simulink model "EcoCAR3_Capstone_P2_LEA_GKN_Enerdel_TheREALone"  (R2014a)
settings: Solver=ode45  StartTime=0.0  StopTime=10.0  RelTol=1e-3
undefined symbols (not defined in the file): chas, DriverControls, EcoCAR3_Lib, eng, eng_plant_init, engine, engine_ratio, env, ENV, fd, gb, gb_ctrl_init, gb_ctrl_trs_init, max_cap, max_cell_curr, motor_ratio, motor_sync_k, motor_sync_Kd, motor_sync_Ki, motor_sync_Kp, num_cell_par, num_cell_series, veh, VEH, veh_plant_init, vpa, vpc, vpc_brake_init, whl, whl_plant_init
libraries: simulink x20
(part 1 of 3)
settings Model: Creator=skumar77  LastModifiedBy=Rashad

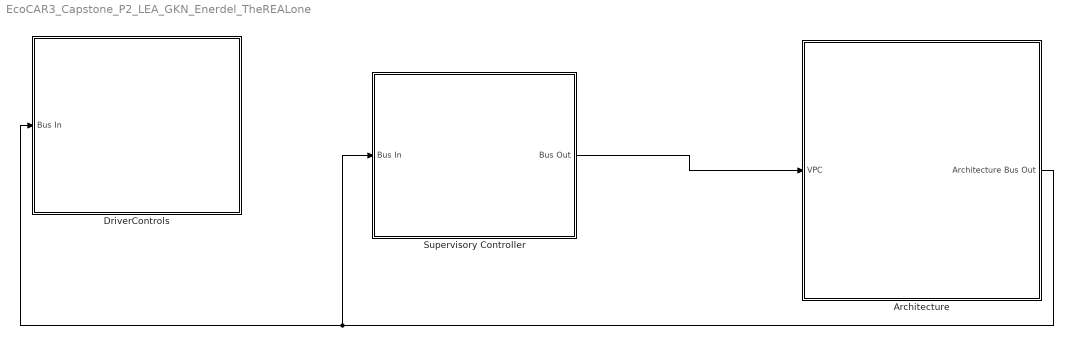
== system EcoCAR3_Capstone_P2_LEA_GKN_Enerdel_TheREALone ==
  Architecture : Subsystem
  DriverControls : Subsystem  AncestorBlock=EcoCAR3_Lib/DriverControls
  Supervisory Controller : Subsystem
  wires:
  Architecture/1(Architecture Bus Out) -> Supervisory Controller/1(Bus In), DriverControls/1(Bus In)
  Supervisory Controller/1(Bus Out) -> Architecture/1(VPC)

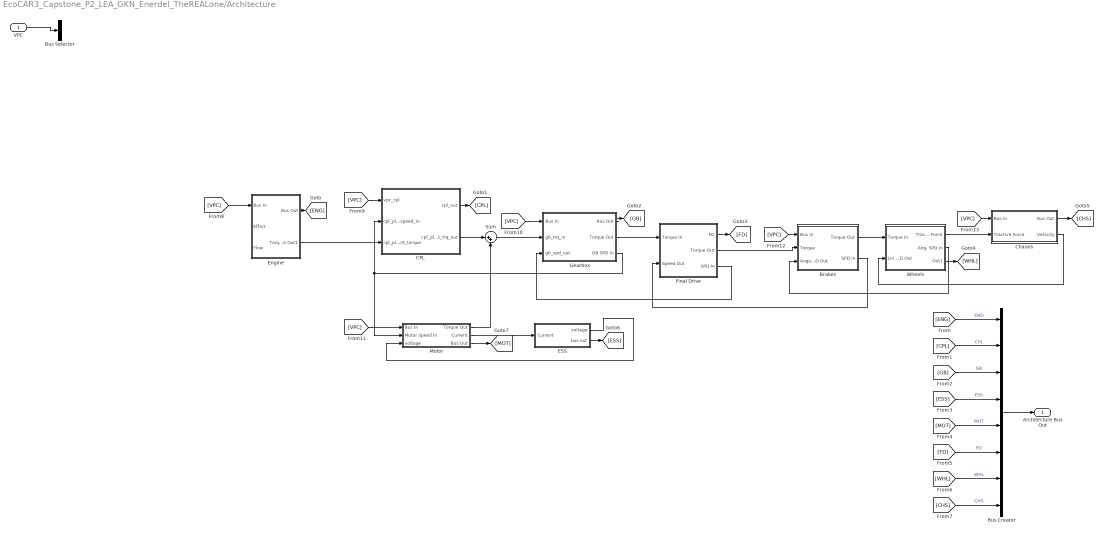
== system EcoCAR3_Capstone_P2_LEA_GKN_Enerdel_TheREALone/Architecture ==
  VPC : Inport
  Brakes : Subsystem
  Bus Creator : BusCreator  Inputs=8
  Bus Selector : BusSelector  OutputSignals=signal1,signal2
  CPL : Subsystem
  Chassis : Subsystem
  ESS : Subsystem
  Engine : Subsystem
  Final Drive : Subsystem
  Gearbox : Subsystem
  Motor : Subsystem
  Sum : Sum  Inputs=|++
  Wheels : Subsystem
  Architecture Bus Out : Outport
  wires:
  Bus Creator/1 -> Architecture Bus Out/1
  [ENG] -> Bus Creator/1  "ENG"
  [CPL] -> Bus Creator/2  "CPL"
  [GB] -> Bus Creator/3  "GB"
  [ESS] -> Bus Creator/4  "ESS"
  [MOT] -> Bus Creator/5  "MOT"
  [FD] -> Bus Creator/6  "FD"
  [WHL] -> Bus Creator/7  "WHL"
  [CHS] -> Bus Creator/8  "CHS"
  Engine/2(Torque Out1) -> CPL/3(cpl_plant_torque)
  Engine/1(Bus Out) -> [ENG]
  Gearbox/3(GB SPD In) -> Motor/2(Motor Speed In), CPL/2(cpl_plant_speed_in)
  Final Drive/3(SPD In) -> Gearbox/3(gb_spd_out)
  Gearbox/2(Torque Out) -> Final Drive/1(Torque In)
  CPL/1(cpl_out) -> [CPL]
  Gearbox/1(Bus Out) -> [GB]
  Final Drive/1(FD) -> [FD]
  CPL/2(cpl_plant_trq_out) -> Sum/1
  Sum/1 -> Gearbox/2(gb_trq_in)
  Motor/1(Torque Out) -> Sum/2
  Final Drive/2(Torque Out) -> Brakes/2(Torque)
  Wheels/2(Ang. SPD In) -> Brakes/3(Angular SPD Out)
  Chassis/2(Velocity) -> Wheels/2(Lin SPD Out)
  Brakes/1(Torque Out) -> Wheels/1(Torque In)
  Brakes/2(SPD In) -> Final Drive/2(Speed Out)
  Wheels/1(Tractive Force) -> Chassis/2(Tractive Force)
  Chassis/1(Bus Out) -> [CHS]
  Motor/2(Current) -> ESS/1(Current)
  ESS/1(voltage) -> Motor/3(voltage)
  Wheels/3(Out1) -> [WHL]
  Motor/3(Bus Out) -> [MOT]
  ESS/2(bus out) -> [ESS]
  [VPC] -> Engine/1(Bus In)
  [VPC] -> CPL/1(vpc_cpl)
  [VPC] -> Gearbox/1(Bus In)
  [VPC] -> Motor/1("Bus In ")
  [VPC] -> Brakes/1(Bus In)
  [VPC] -> Chassis/1(Bus In)
  VPC/1 -> Bus Selector/1

== system EcoCAR3_Capstone_P2_LEA_GKN_Enerdel_TheREALone/DriverControls ==
  Bus In : Inport
  Bus Selector : BusSelector  OutputSignals=CHS
  Driver : Subsystem
  Velocity Profile : Subsystem
  wires:
  Bus Selector/1 -> Driver/2(Measured Velocity)  "<CHS>"
  Velocity Profile/1(Out1) -> Driver/1(Commanded Velocity)
  Bus In/1 -> Bus Selector/1

== system EcoCAR3_Capstone_P2_LEA_GKN_Enerdel_TheREALone/Supervisory Controller ==
  Bus In : Inport
  Brake : Subsystem  Commented=on
  ComponentDiag : Subsystem
  SignalDiag : Subsystem
  Subsystem : Subsystem  Commented=on
  SupervisoryControl : Subsystem
  System Diag : Subsystem
  vpc_prop_par_direct_pwr_1mot_pretx : Subsystem  Commented=on
  Bus Out : Outport
  wires:
  Bus In/1 -> SignalDiag/1(In1)
  SignalDiag/1(Out1) -> ComponentDiag/1(In1)
  ComponentDiag/1(Out1) -> System Diag/1(In1)
  System Diag/1(Out1) -> SupervisoryControl/1(In1)
  SupervisoryControl/1(Out1) -> Bus Out/1

== system EcoCAR3_Capstone_P2_LEA_GKN_Enerdel_TheREALone/Architecture/Brakes ==
  Bus In : Inport
  Torque : Inport  Port=2
  Angular SPD Out : Inport  Port=3
  Plant : Subsystem
  Torque Out : Outport
  SPD In : Outport  Port=2
  wires:
  Torque/1 -> Plant/2(Torque In)
  Angular SPD Out/1 -> Plant/3(Angular Speed Out)
  Plant/2(Angular Speed In) -> SPD In/1
  Plant/1(Torque Out) -> Torque Out/1
  Bus In/1 -> Plant/1(Brake CMD)

== system EcoCAR3_Capstone_P2_LEA_GKN_Enerdel_TheREALone/Architecture/CPL ==
  vpc_cpl : Inport
  cpl_plant_speed_in : Inport  Port=2
  cpl_plant_torque : Inport  Port=3
  Bus Creator : BusCreator  Inputs=2
  Bus Selector : BusSelector  OutputSignals=signal2.cpl_plant_trq_out
  Ctrl : Subsystem
  Plant : Subsystem
  cpl_out : Outport
  cpl_plant_trq_out : Outport  Port=2
  wires:
  Bus Creator/1 -> Bus Selector/1, cpl_out/1
  [PLNT] -> Bus Creator/2
  [CTRL] -> Bus Creator/1
  vpc_cpl/1 -> Ctrl/1(vpc_cpl)
  Ctrl/1(cpl_ctrl_command) -> Plant/1(cpl_command), [CTRL]
  Plant/1(cpl_plant_out) -> [PLNT]
  cpl_plant_torque/1 -> Plant/2(cpl_torque)
  Bus Selector/1 -> cpl_plant_trq_out/1  "<cpl_plant_trq_out>"
  cpl_plant_speed_in/1 -> Plant/3(cpl_speed)

== system EcoCAR3_Capstone_P2_LEA_GKN_Enerdel_TheREALone/Architecture/Chassis ==
  Bus In : Inport
  Tractive Force : Inport  Port=2
  Plant : Subsystem
  Bus Out : Outport
  Velocity : Outport  Port=2
  wires:
  Plant/1(Velocity) -> Velocity/1
  Tractive Force/1 -> Plant/1(Tractive Force)
  Bus In/1 -> Plant/2(Accelerator Position)
  Plant/2(Bus Out) -> Bus Out/1

== system EcoCAR3_Capstone_P2_LEA_GKN_Enerdel_TheREALone/Architecture/ESS ==
  Current : Inport
  Bus Creator : BusCreator  Inputs=3
  Bus Creator1 : BusCreator
  Bus Creator2 : BusCreator  Inputs=2
  Plant : Subsystem
  ess_controller_PI : Subsystem
  voltage : Outport
  bus out : Outport  Port=2
  wires:
  Current/1 -> Bus Creator/1, Plant/1(Current)  "current"
  Plant/2(voltage) -> Bus Creator/2, voltage/1  "voltage"
  Bus Creator/1 -> ess_controller_PI/1(In1)
  ess_controller_PI/4(current_max_reg) -> Bus Creator1/4
  ess_controller_PI/3(power_max_reg) -> Bus Creator1/3
  ess_controller_PI/2(current_max_prop) -> Bus Creator1/2
  ess_controller_PI/1(power_max_prop) -> Bus Creator1/1
  Plant/1("SOC ") -> Bus Creator/3, Bus Creator2/1  "soc"
  Plant/3(bus out) -> Bus Creator2/2
  Bus Creator2/1 -> bus out/1

== system EcoCAR3_Capstone_P2_LEA_GKN_Enerdel_TheREALone/Architecture/Engine ==
  Bus In : Inport
  Effort : Inport  Port=2
  Flow : Inport  Port=3
  Bus Creator : BusCreator  Inputs=2
  Bus Selector : BusSelector  OutputSignals=signal1,signal2
  Controller : Subsystem
  Plant1 : Subsystem
  Bus Out : Outport
  Torque Out1 : Outport  Port=2
  wires:
  Bus Creator/1 -> Bus Out/1
  [CTRL] -> Bus Creator/1  "CTRL"
  [PLNT] -> Bus Creator/2  "PLT"
  Bus In/1 -> Bus Selector/1
  Plant1/1(Bus Out) -> [PLNT]
  Plant1/2(Torque Out) -> Torque Out1/1
  Flow/1 -> Plant1/1(Engine Speed)

== system EcoCAR3_Capstone_P2_LEA_GKN_Enerdel_TheREALone/Architecture/Final Drive ==
  Torque In : Inport
  Speed Out : Inport  Port=2
  Bus Creator : BusCreator  Inputs=1
  Bus Creator1 : BusCreator  Inputs=2
  Plant : Subsystem
  FD : Outport
  Torque Out : Outport  Port=2
  SPD In : Outport  Port=3
  wires:
  Speed Out/1 -> Plant/1(FD SPD Out)
  Torque In/1 -> Plant/2(FD Torque In)
  Plant/1(SPD In) -> Bus Creator1/1, SPD In/1  "gb_plant_spd_in"
  Plant/2(Torque Out) -> Bus Creator1/2, Torque Out/1  "gb_plant_trq_out"
  Bus Creator/1 -> FD/1
  [PLNT] -> Bus Creator/1
  Bus Creator1/1 -> [PLNT]

== system EcoCAR3_Capstone_P2_LEA_GKN_Enerdel_TheREALone/Architecture/Gearbox ==
  Bus In : Inport
  gb_trq_in : Inport  Port=2
  gb_spd_out : Inport  Port=3
  Bus Creator : BusCreator  Inputs=2
  Bus Creator1 : BusCreator  Inputs=2
  Controller : Subsystem
  Plant : Subsystem
  Bus Out : Outport
  Torque Out : Outport  Port=2
  GB SPD In : Outport  Port=3
  wires:
  Controller/1(Out1) -> Plant/3(Gear CMD), [CTRL]
  gb_spd_out/1 -> Plant/1(GB SPD Out)
  gb_trq_in/1 -> Plant/2(GB Torque in)
  Plant/1(GB SPD In) -> Bus Creator1/1, GB SPD In/1  "gb_plant_spd_in"
  Bus Creator/1 -> Bus Out/1
  [CTRL] -> Bus Creator/2
  [PLNT] -> Bus Creator/1
  Plant/2(GB Torque Out) -> Bus Creator1/2, Torque Out/1  "gb_trq_out"
  Bus Creator1/1 -> [PLNT]
  Bus In/1 -> Controller/1(In1)

== system EcoCAR3_Capstone_P2_LEA_GKN_Enerdel_TheREALone/Architecture/Motor ==
  "Bus In " : Inport
  Motor Speed In : Inport  Port=2
  voltage : Inport  Port=3
  Bus Creator : BusCreator  Inputs=2
  Controller : Subsystem
  Plant : Subsystem
  Torque Out : Outport
  Current : Outport  Port=2
  Bus Out : Outport  Port=3
  wires:
  Controller/1(Out1) -> Plant/2(Torque CMD %)
  Motor Speed In/1 -> Plant/1(Motor Speed)
  "Bus In "/1 -> Controller/1(In1)
  Plant/2(Current) -> Current/1
  Plant/1(Torque Out) -> Torque Out/1
  voltage/1 -> Plant/3(voltage)
  [CTRL] -> Bus Creator/2  "CTRL"
  [PLNT] -> Bus Creator/1  "PLNT"
  Bus Creator/1 -> Bus Out/1
  Plant/3(motor_plnt) -> [PLNT]
  Controller/2(bus out) -> [CTRL]

== system EcoCAR3_Capstone_P2_LEA_GKN_Enerdel_TheREALone/Architecture/Wheels ==
  Torque In : Inport
  Lin SPD Out : Inport  Port=2
  Bus Creator : BusCreator  Inputs=2
  Plant : Subsystem
  Tractive Force : Outport
  Ang. SPD In : Outport  Port=2
  Out1 : Outport  Port=3
  wires:
  Torque In/1 -> Plant/1(Wheel Torque)
  Lin SPD Out/1 -> Plant/2(Linear Speed in)
  Plant/1(Tractive Force) -> Bus Creator/1, Tractive Force/1  "whl_plant_tractiveforce"
  Plant/2(Angular Speed) -> Bus Creator/2, Ang. SPD In/1  "whl_plant_speed"
  Bus Creator/1 -> Out1/1

== system EcoCAR3_Capstone_P2_LEA_GKN_Enerdel_TheREALone/DriverControls/Driver ==
  Commanded Velocity : Inport
  Measured Velocity : Inport  Port=2
  BrakeForce : Gain  Gain=5000
  Gain : Gain  Gain=-1
  Memory : Memory
  Memory1 : Memory
  PID Controller : simulink/Continuous/PID Controller  Controller=PI  TimeDomain=Continuous-time  SampleTime=1  IntegratorMethod=Forward Euler  FilterMethod=Forward Euler  Form=Parallel  P=.2  I=.004  D=0  N=100  InitialConditionSource=internal  InitialConditionForIntegrator=0  InitialConditionForFilter=0  ExternalReset=none  LimitOutput=on  UpperSaturationLimit=1  LowerSaturationLimit=-5  LinearizeAsGain=on  AntiWindupMode=clamping  Kb=1  TrackingMode=off  Kt=1  PParamMin=[]  PParamMax=[]  IParamMin=[]  IParamMax=[]  DParamMin=[]  DParamMax=[]  NParamMin=[]  NParamMax=[]  KbParamMin=[]  KbParamMax=[]  KtParamMin=[]  KtParamMax=[]  POutMin=[]  POutMax=[]  IOutMin=[]  IOutMax=[]  DOutMin=[]  DOutMax=[]  NOutMin=[]  NOutMax=[]  KbOutMin=[]  KbOutMax=[]  KtOutMin=[]  KtOutMax=[]  IntegratorOutMin=[]  IntegratorOutMax=[]  FilterOutMin=[]  FilterOutMax=[]  SumOutMin=[]  SumOutMax=[]  SumI1OutMin=[]  SumI1OutMax=[]  SumI2OutMin=[]  SumI2OutMax=[]  SumI3OutMin=[]  SumI3OutMax=[]  SumDOutMin=[]  SumDOutMax=[]  SaturationOutMin=[]  SaturationOutMax=[]  IntegratorContinuousStateAttributes=''  IntegratorStateMustResolveToSignalObject=off  IntegratorRTWStateStorageClass=Auto  FilterContinuousStateAttributes=''  FilterStateMustResolveToSignalObject=off  FilterRTWStateStorageClass=Auto
  Pct : Gain  Gain=100
  Saturation : Saturate  UpperLimit=1  LowerLimit=0
  Saturation1 : Saturate  UpperLimit=0  LowerLimit=-1
  Sum1 : Sum  Inputs=+-|
  Brake : Outport
  Accelerator Position : Outport  Port=2
  wires:
  Commanded Velocity/1 -> Sum1/2
  Sum1/1 -> PID Controller/1
  Measured Velocity/1 -> Sum1/1
  Pct/1 -> Memory1/1
  Memory/1 -> Brake/1
  Memory1/1 -> Accelerator Position/1
  BrakeForce/1 -> Memory/1
  Saturation/1 -> BrakeForce/1
  PID Controller/1 -> Saturation/1, Saturation1/1
  Saturation1/1 -> Gain/1
  Gain/1 -> Pct/1

== system EcoCAR3_Capstone_P2_LEA_GKN_Enerdel_TheREALone/DriverControls/Velocity Profile ==
  DriveCycle Select : Subsystem  AncestorBlock=EcoCAR3_Lib/DriveCycle Select  mask(Drive Cycle){Drive_Cycle_Num=EcoCAR city 1}
      mask prompts: Drive_Cycle_Num "Select the desired drive cycle"
      mask help:
      | Select the drive cycle you wish to input to the vehicle model.
      | The simulation run time and assertions will be updated accordingly.
      settings: AttributesFormatString=%<Drive_Cycle_Num> (kph)
      mask TypeOptions Drive_Cycle_Num: EcoCAR city 1 | EcoCAR city 2 | EcoCAR hwy | FTP75 | Cruise Mode | US06
      mask Callback Drive_Cycle_Num:
      | maskStr = get_param(gcb,'MaskValues');
      | maskStr = maskStr{1};
      | mdnm = get_param(gcs,'Name');
      | % Urban 1
      | % Urban 2
      | % Urban 3
      | % Urban 4
      | % FTP75
      | % US06
      | % Combined 0-60, FTP75
      | % Combined 0-60, US06
      | switch maskStr
      |     case 'Urban 1'
      |         setsim(1,200,mdnm);
      |         zero2sixty_cuttoff_time = inf;
      |     case 'Urban 2'
      |         setsim(2,200,mdnm);
      |         zero2sixty_cuttoff_time = inf;
      |     case 'Urban 3'
      |         setsim(3,200,mdnm);
      |         zero2sixty_cuttoff_time = inf;
      |     case 'FTP75'
      |         setsim(4,490,mdnm);
      |         zero2sixty_cuttoff_time = inf;
      |     case 'Cruise Mode'
      |         setsim(5,129,mdnm);
      |         zero2sixty_cuttoff_time = inf;
      |     case 'US06'
      |         setsim(6,600,mdnm);
      |         zero2sixty_cuttoff_time = inf;
      |     case 'Combined 0-60, FTP75'
      |         setsim(7,650,mdnm);
      |         zero2sixty_cuttoff_time = 15;
      |     case 'Combined 0-60, US06'
      |         setsim(8,650,mdnm);
      |         zero2sixty_cuttoff_time = 15;
      |     otherwise
      |         setsim(8,650,mdnm);
      |         zero2sixty_cuttoff_time = 15;
      | end
      | 
      | % function setsim(caseno,simtime,modelname)
      | %      assignin('base','Drive_Cycle_Num',caseno);
      | %      evalin('base',['set_param(''' modelname ''',''StartTime'',''0'',''StopTime'',''' num2str(simtime) ''') ';'']);
      | %      %eval(['set_param(''' modelname ''',''StartTime'',''0'',''StopTime'',''' num2str(simtime) ''') ';'']);
      | % end
  Subsystem : Subsystem  mask(Select Mode){Choice=DriveCycle Select}
      mask prompts: Choice "Select mode"
      mask help: Select acceleration, braking or drive cycle execution mode
      mask TypeOptions Choice: acceleration test | brake test | DriveCycle Select
  acceleration test : FromWorkspace  VariableName=[acc.time acc.SpdKph]  SampleTime=0
  brake test : FromWorkspace  VariableName=[brake.time brake.SpdKph]  SampleTime=0
  Out1 : Outport
  wires:
  DriveCycle Select/1(kph) -> Subsystem/3(In3)
  brake test/1 -> Subsystem/2(In2)
  acceleration test/1 -> Subsystem/1(In1)
  Subsystem/1(Out1) -> Out1/1  "Velocity Profile"

== system EcoCAR3_Capstone_P2_LEA_GKN_Enerdel_TheREALone/Supervisory Controller/Brake ==
  drv_brk_cmd : Inport
  chas_spd : Inport  Port=2
  ess_soc : Inport  Port=3
  gb_gear_ratio : Inport  Port=4
  gb_gear_sft_in_progress : Inport  Port=5
  cpl_cmd : Inport  Port=6
  mot_main_spd : Inport  Port=7
  ess_pwr_max_neg : Inport  Port=8
  mot_main_trq_max : Inport  Port=9
  Brake ECU Torque : Subsystem
  Chassis speed ESS SOC limits : Subsystem
  Electric power available : Subsystem
  Gear shifting : Subsystem
  Main motor brake torque demand : Subsystem
  Motor main torque max : Subsystem
  Saturation : Saturate  UpperLimit=0  LowerLimit=-inf
  Sum : Sum  Inputs=+-
  Terminator : Terminator
  Terminator1 : Terminator
  "Torque demand at wheels " : Subsystem
  whl_brk_trq_ECU_dmd : Outport
  mot_main_trq_dmd : Outport  Port=2
  wires:
  drv_brk_cmd/1 -> "Torque demand at wheels "/1(brake_signal_dmd)
  "Torque demand at wheels "/1(whl_trq_dmd) -> Brake ECU Torque/1(whl_trq_dmd)
  Brake ECU Torque/2(whl_twr_brk_ECU) -> Chassis speed ESS SOC limits/1(whl_trq_brake_ECU), Sum/1
  Brake ECU Torque/1(whl_twr_brk_emergency) -> Terminator/1
  Sum/1 -> Saturation/1
  Saturation/1 -> whl_brk_trq_ECU_dmd/1
  ess_soc/1 -> Chassis speed ESS SOC limits/3(ess_soc)
  Chassis speed ESS SOC limits/1(whl_trq_regen_available) -> Main motor brake torque demand/1(whl_trq_regen_max)
  Main motor brake torque demand/1(mot_trq_dmd) -> mot_main_trq_dmd/1
  Main motor brake torque demand/3(mot_pwr_elec_estimated) -> Terminator1/1
  Main motor brake torque demand/2(mot_trq_dmd_at_wheels) -> Sum/2
  gb_gear_ratio/1 -> Gear shifting/1(gb_gear_ratio)
  gb_gear_sft_in_progress/1 -> Gear shifting/2(gb_sft_in_progress)
  cpl_cmd/1 -> Gear shifting/3(cpl_cmd)
  Gear shifting/1(gear_ratio) -> Main motor brake torque demand/2(ratio_gear)
  Gear shifting/2(coeff_mult_gear) -> Main motor brake torque demand/3(coef_mult_sft)
  ess_pwr_max_neg/1 -> Electric power available/1(ess_pwr_max_neg)
  Electric power available/1(pwr_elec_available_regen) -> Motor main torque max/2(pwr_elec_max)
  mot_main_spd/1 -> Motor main torque max/1(mot_spd), Main motor brake torque demand/4(mot_spd)
  mot_main_trq_max/1 -> Motor main torque max/3(mot_trq_max)
  Motor main torque max/1(mot_trq_maximum) -> Main motor brake torque demand/5(mot_trq_max_regen)
  chas_spd/1 -> Chassis speed ESS SOC limits/2(chas_spd)

== system EcoCAR3_Capstone_P2_LEA_GKN_Enerdel_TheREALone/Supervisory Controller/ComponentDiag ==
  In1 : Inport
  Bus Creator{,1..5} (6 alike) : BusCreator  Inputs=2
  Bus Selector{,1..5} (6 alike) : BusSelector  OutputSignals=signal1,signal2
  Out1 : Outport
  wires:
  In1/1 -> Bus Selector5/1, Bus Selector4/1, Bus Selector3/1, Bus Selector2/1, Bus Selector1/1, Bus Selector/1

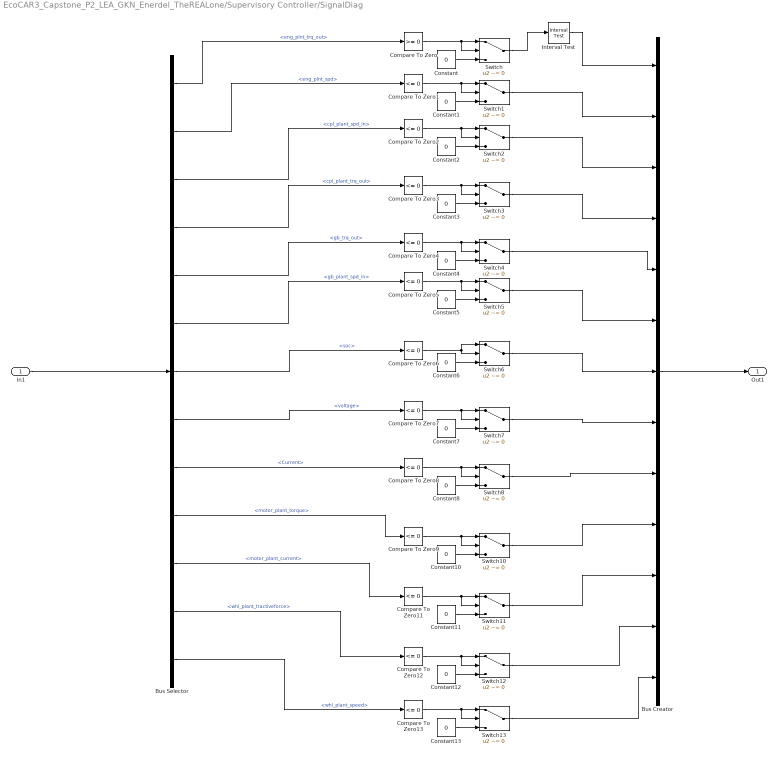
== system EcoCAR3_Capstone_P2_LEA_GKN_Enerdel_TheREALone/Supervisory Controller/SignalDiag ==
  In1 : Inport
  Bus Creator : BusCreator  Inputs=13
  Bus Selector : BusSelector  OutputSignals=ENG.PLT.eng_plnt_trq_out,ENG.PLT.eng_plnt_spd,CPL.signal2.cpl_plant_spd_in,CPL.signal2.cpl_plant_trq_out,GB.signal1.gb_trq_out,GB.signal1.gb_plant_spd_in,ESS.soc,ESS.signal2.voltage,ESS.signal2.Current,MOT.PLNT.motor_plant_torque,MOT.PLNT.motor_plant_current,WHL.whl_plant_tractiveforce,WHL.whl_plant_speed
  Compare To Zero : simulink/Logic and Bit Operations/Compare To Zero  relop=>=  OutDataTypeStr=boolean
  Compare To Zero{1..9,11..13} (12 alike) : simulink/Logic and Bit Operations/Compare To Zero  relop=<=  OutDataTypeStr=boolean
  Constant{,1..8,10..13} (13 alike) : Constant  Value=0
  Interval Test : simulink/Logic and Bit Operations/Interval Test  IntervalClosedRight=on  uplimit=0.5  IntervalClosedLeft=on  lowlimit=-0.5  OutDataTypeStr=boolean
  Switch{,1..8,10..13} (13 alike) : Switch  Criteria=u2 ~= 0
  Out1 : Outport
  wires:
  In1/1 -> Bus Selector/1
  Bus Creator/1 -> Out1/1
  Compare To Zero/1 -> Switch/2, Switch/1
  Constant/1 -> Switch/3
  Compare To Zero1/1 -> Switch1/1, Switch1/2
  Constant1/1 -> Switch1/3
  Compare To Zero2/1 -> Switch2/2, Switch2/1
  Constant2/1 -> Switch2/3
  Compare To Zero3/1 -> Switch3/1, Switch3/2
  Constant3/1 -> Switch3/3
  Compare To Zero4/1 -> Switch4/2, Switch4/1
  Constant4/1 -> Switch4/3
  Compare To Zero5/1 -> Switch5/1, Switch5/2
  Constant5/1 -> Switch5/3
  Compare To Zero6/1 -> Switch6/1, Switch6/2
  Constant6/1 -> Switch6/3
  Compare To Zero7/1 -> Switch7/1, Switch7/2
  Constant7/1 -> Switch7/3
  Compare To Zero8/1 -> Switch8/2, Switch8/1
  Constant8/1 -> Switch8/3
  Compare To Zero9/1 -> Switch10/2, Switch10/1
  Constant10/1 -> Switch10/3
  Compare To Zero11/1 -> Switch11/1, Switch11/2
  Constant11/1 -> Switch11/3
  Compare To Zero12/1 -> Switch12/2, Switch12/1
  Constant12/1 -> Switch12/3
  Compare To Zero13/1 -> Switch13/1, Switch13/2
  Constant13/1 -> Switch13/3
  Bus Selector/13 -> Compare To Zero13/1  "<whl_plant_speed>"
  Bus Selector/12 -> Compare To Zero12/1  "<whl_plant_tractiveforce>"
  Bus Selector/11 -> Compare To Zero11/1  "<motor_plant_current>"
  Bus Selector/10 -> Compare To Zero9/1  "<motor_plant_torque>"
  Bus Selector/9 -> Compare To Zero8/1  "<Current>"
  Bus Selector/8 -> Compare To Zero7/1  "<voltage>"
  Bus Selector/7 -> Compare To Zero6/1  "<soc>"
  Bus Selector/6 -> Compare To Zero5/1  "<gb_plant_spd_in>"
  Bus Selector/5 -> Compare To Zero4/1  "<gb_trq_out>"
  Bus Selector/4 -> Compare To Zero3/1  "<cpl_plant_trq_out>"
  Bus Selector/3 -> Compare To Zero2/1  "<cpl_plant_spd_in>"
  Bus Selector/2 -> Compare To Zero1/1  "<eng_plnt_spd>"
  Bus Selector/1 -> Compare To Zero/1  "<eng_plnt_trq_out>"
  Switch8/1 -> Bus Creator/9
  Switch7/1 -> Bus Creator/8
  Switch6/1 -> Bus Creator/7
  Switch5/1 -> Bus Creator/6
  Switch4/1 -> Bus Creator/5
  Switch3/1 -> Bus Creator/4
  Switch2/1 -> Bus Creator/3
  Switch1/1 -> Bus Creator/2
  Switch/1 -> Interval Test/1
  Switch10/1 -> Bus Creator/10
  Switch11/1 -> Bus Creator/11
  Switch12/1 -> Bus Creator/12
  Switch13/1 -> Bus Creator/13
  Interval Test/1 -> Bus Creator/1

== system EcoCAR3_Capstone_P2_LEA_GKN_Enerdel_TheREALone/Supervisory Controller/Subsystem ==
  Eng : Inport
  ESS : Inport  Port=2
  CPL : Inport  Port=3
  Motor : Inport  Port=4
  GB : Inport  Port=5
  FD : Inport  Port=6
  WHL : Inport  Port=7
  CHS : Inport  Port=8
  Key pos : Inport  Port=9
  Constant : Constant  Value=0
  Rate Limiter2 : RateLimiter  RisingSlewLimit=250  FallingSlewLimit=-250  SampleTimeMode=inherited
  SupervisoryLogicChart : Stateflow chart  TreatAsAtomicUnit=on
  VPC Eng : Outport
  "VPC CPL " : Outport  Port=2
  VPC motor : Outport  Port=3
  VPC GB : Outport  Port=4
  VPC Brakes : Outport  Port=5
  VPC CHS : Outport  Port=6
  wires:
  ? -> SupervisoryLogicChart/1(eSystemStatus)  "<eSystemStatus>"
  ? -> SupervisoryLogicChart/3(APP_percent)  "<APP [%]>"
  ? -> SupervisoryLogicChart/4(BPP_percent)  "<BPP [%]>"
  ? -> SupervisoryLogicChart/5(keyPos)  "< keyPos [0_3]>"
  SupervisoryLogicChart/1(motTrqReq_percent) -> Rate Limiter2/1
  SupervisoryLogicChart/7(ChartMode) -> ?
  ? -> SupervisoryLogicChart/6(vehVel_mph)  "<vehVel [mph]>"
  SupervisoryLogicChart/3(hydBrkReq_percent) -> ?
  ? -> SupervisoryLogicChart/7(regenFactor)  "<regenFactor>"
  ? -> ?  "<PRNDL>"
  SupervisoryLogicChart/2(engTrqReq_percent) -> ?
  SupervisoryLogicChart/4(powerMode) -> ?
  SupervisoryLogicChart/5(closeContactorsReq) -> ?
  SupervisoryLogicChart/6(engOnReq) -> ?
  ? -> SupervisoryLogicChart/2(iceSystemStatus)  "<iceSystemStatus>"
  Rate Limiter2/1 -> ?  "motTrqReq_percent"
  Constant/1 -> SupervisoryLogicChart/9(motDrag_percent)
  ? -> SupervisoryLogicChart/8(essSOC_0_1)  "<essSOC_0_1>"

== system EcoCAR3_Capstone_P2_LEA_GKN_Enerdel_TheREALone/Supervisory Controller/SupervisoryControl ==
  In1 : Inport
  Bus Creator : BusCreator  Inputs=2
  Bus Selector : BusSelector  OutputSignals=signal1,signal2
  SupervisorLogic : Stateflow chart  TreatAsAtomicUnit=on
  Out1 : Outport
  wires:
  In1/1 -> Bus Selector/1
  Bus Creator/1 -> Out1/1

== system EcoCAR3_Capstone_P2_LEA_GKN_Enerdel_TheREALone/Supervisory Controller/System Diag ==
  In1 : Inport
  Bus Creator{,1..3} (4 alike) : BusCreator  Inputs=2
  Bus Selector{,1..3} (4 alike) : BusSelector  OutputSignals=signal1,signal2
  Out1 : Outport

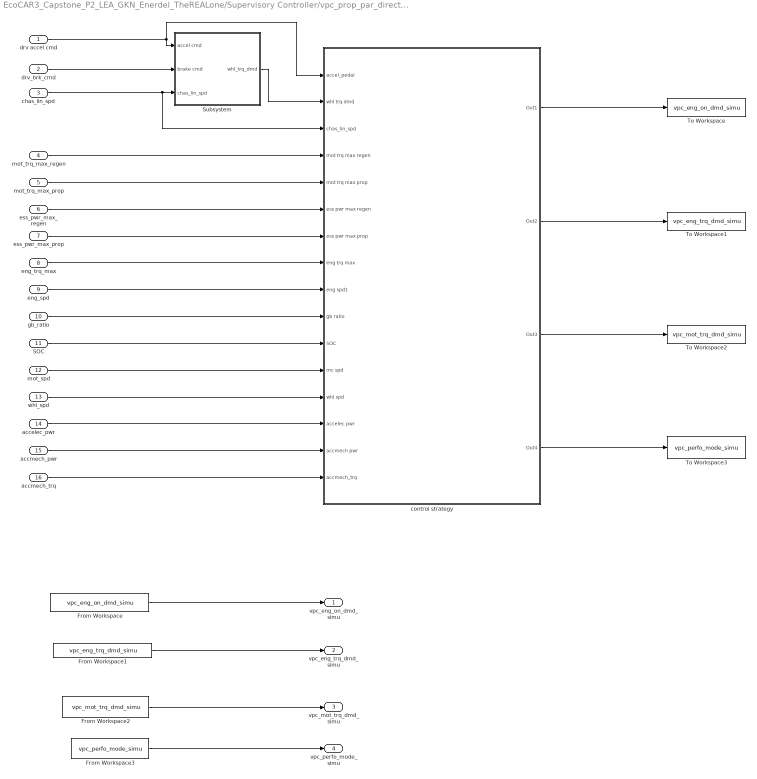
== system EcoCAR3_Capstone_P2_LEA_GKN_Enerdel_TheREALone/Supervisory Controller/vpc_prop_par_direct_pwr_1mot_pretx ==
  drv accel cmd : Inport
  drv_brk_cmd : Inport  Port=2
  chas_lin_spd : Inport  Port=3
  mot_trq_max_regen : Inport  Port=4
  mot_trq_max_prop : Inport  Port=5
  ess_pwr_max_regen : Inport  Port=6
  ess_pwr_max_prop : Inport  Port=7
  eng_trq_max : Inport  Port=8
  eng_spd : Inport  Port=9
  gb_ratio : Inport  Port=10
  SOC : Inport  Port=11
  mot_spd : Inport  Port=12
  whl_spd : Inport  Port=13
  accelec_pwr : Inport  Port=14
  accmech_pwr : Inport  Port=15
  accmech_trq : Inport  Port=16
  From Workspace : FromWorkspace  VariableName=vpc_eng_on_dmd_simu  SampleTime=0
  From Workspace1 : FromWorkspace  VariableName=vpc_eng_trq_dmd_simu  SampleTime=0
  From Workspace2 : FromWorkspace  VariableName=vpc_mot_trq_dmd_simu  SampleTime=0
  From Workspace3 : FromWorkspace  VariableName=vpc_perfo_mode_simu  SampleTime=0
  Subsystem : Subsystem
  To Workspace : ToWorkspace  VariableName=vpc_eng_on_dmd_simu  SaveFormat=Timeseries  SampleTime=-1
  To Workspace1 : ToWorkspace  VariableName=vpc_eng_trq_dmd_simu  SaveFormat=Timeseries  SampleTime=-1
  To Workspace2 : ToWorkspace  VariableName=vpc_mot_trq_dmd_simu  SaveFormat=Timeseries  SampleTime=-1
  To Workspace3 : ToWorkspace  VariableName=vpc_perfo_mode_simu  SaveFormat=Timeseries  SampleTime=-1
  control strategy : Subsystem
  vpc_eng_on_dmd_simu : Outport
  vpc_eng_trq_dmd_simu : Outport  Port=2
  vpc_mot_trq_dmd_simu : Outport  Port=3
  vpc_perfo_mode_simu : Outport  Port=4
  wires:
  From Workspace2/1 -> vpc_mot_trq_dmd_simu/1
  From Workspace1/1 -> vpc_eng_trq_dmd_simu/1
  From Workspace/1 -> vpc_eng_on_dmd_simu/1
  From Workspace3/1 -> vpc_perfo_mode_simu/1
  drv_brk_cmd/1 -> Subsystem/2(brake cmd)
  chas_lin_spd/1 -> control strategy/3(chas_lin_spd), Subsystem/3(chas_lin_spd)
  drv accel cmd/1 -> Subsystem/1(accel cmd), control strategy/1(accel_pedal)
  Subsystem/1(whl_trq_dmd) -> control strategy/2(whl trq dmd)
  mot_trq_max_regen/1 -> control strategy/4(mot trq max regen)
  mot_trq_max_prop/1 -> control strategy/5(mot trq max prop)
  accmech_trq/1 -> control strategy/16(accmech_trq)
  accmech_pwr/1 -> control strategy/15(accmech pwr)
  accelec_pwr/1 -> control strategy/14(accelec pwr)
  whl_spd/1 -> control strategy/13(whl spd)
  ess_pwr_max_regen/1 -> control strategy/6(ess pwr max regen)
  ess_pwr_max_prop/1 -> control strategy/7(ess pwr max prop)
  eng_trq_max/1 -> control strategy/8(eng trq max)
  eng_spd/1 -> control strategy/9(eng spd1)
  gb_ratio/1 -> control strategy/10(gb ratio)
  SOC/1 -> control strategy/11(SOC)
  mot_spd/1 -> control strategy/12(mc spd)
  control strategy/4(Out4) -> To Workspace3/1
  control strategy/3(Out3) -> To Workspace2/1
  control strategy/2(Out2) -> To Workspace1/1
  control strategy/1(Out1) -> To Workspace/1

== system EcoCAR3_Capstone_P2_LEA_GKN_Enerdel_TheREALone/Architecture/Brakes/Plant ==
  Brake CMD : Inport
  Torque In : Inport  Port=2
  Angular Speed Out : Inport  Port=3
  Max Brake Force : Constant  Value=whl.brake.max_force
  Product : Product
  Subtract : Sum  Inputs=-+
  Torque Out : Outport
  Angular Speed In : Outport  Port=2
  wires:
  Angular Speed Out/1 -> Angular Speed In/1
  Max Brake Force/1 -> Product/2
  Product/1 -> Subtract/1
  Subtract/1 -> Torque Out/1
  Brake CMD/1 -> Product/1
  Torque In/1 -> Subtract/2

== system EcoCAR3_Capstone_P2_LEA_GKN_Enerdel_TheREALone/Architecture/CPL/Ctrl ==
  vpc_cpl : Inport
  Constant1 : Constant
  Constant2 : Constant  Value=0
  Index Vector : MultiPortSwitch  DataPortOrder=Zero-based contiguous  zeroidx=on
  Rate Limiter : RateLimiter  RisingSlewLimit=2.5  SampleTimeMode=inherited
  Saturation : Saturate  UpperLimit=1  LowerLimit=0
  cpl_ctrl_command : Outport
  wires:
  Index Vector/1 -> cpl_ctrl_command/1
  vpc_cpl/1 -> Index Vector/1, Rate Limiter/1
  Saturation/1 -> Index Vector/4
  Constant2/1 -> Index Vector/2
  Constant1/1 -> Index Vector/3
  Rate Limiter/1 -> Saturation/1

== system EcoCAR3_Capstone_P2_LEA_GKN_Enerdel_TheREALone/Architecture/CPL/Plant ==
  cpl_command : Inport
  cpl_torque : Inport  Port=2
  cpl_speed : Inport  Port=3
  Bus Creator : BusCreator  Inputs=2
  Product : Product
  Product1 : Product
  cpl_plant_out : Outport
  wires:
  cpl_torque/1 -> Product1/2
  cpl_command/1 -> Product1/1, Product/2
  Product1/1 -> Bus Creator/2  "cpl_plant_trq_out"
  Product/1 -> Bus Creator/1  "cpl_plant_spd_in"
  Bus Creator/1 -> cpl_plant_out/1
  cpl_speed/1 -> Product/1

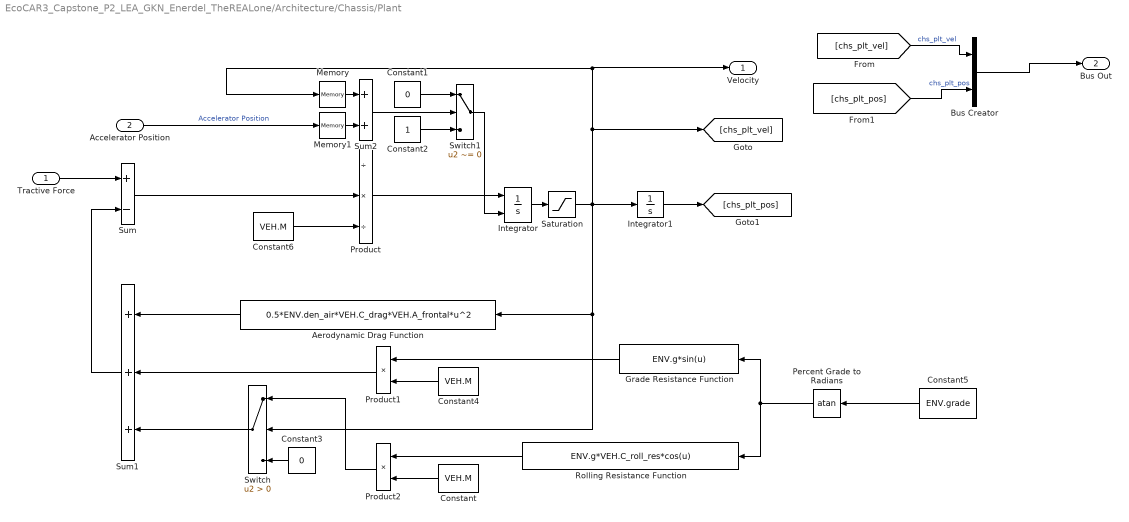
== system EcoCAR3_Capstone_P2_LEA_GKN_Enerdel_TheREALone/Architecture/Chassis/Plant ==
  Tractive Force : Inport
  Accelerator Position : Inport  Port=2
  Aerodynamic Drag Function : Fcn  Expr=0.5*ENV.den_air*VEH.C_drag*VEH.A_frontal*u^2
  Bus Creator : BusCreator  Inputs=2
  Constant : Constant  Value=VEH.M
  Constant1 : Constant  Value=0
  Constant2 : Constant
  Constant3 : Constant  Value=0
  Constant4 : Constant  Value=VEH.M
  Constant5 : Constant  Value=ENV.grade
  Constant6 : Constant  Value=VEH.M
  Grade Resistance Function : Fcn  Expr=ENV.g*sin(u)
  Integrator : Integrator  ExternalReset=level  LowerSaturationLimit=0
  Integrator1 : Integrator
  Memory : Memory
  Memory1 : Memory
  Percent Grade to Radians : Trigonometry  Operator=atan
  Product : Product  Inputs=/*/  RndMeth=Zero
  Product1 : Product  Inputs=**  RndMeth=Zero
  Product2 : Product  Inputs=**  RndMeth=Zero
  Rolling Resistance Function : Fcn  Expr=ENV.g*VEH.C_roll_res*cos(u)
  Saturation : Saturate  UpperLimit=inf  LowerLimit=0
  Sum : Sum  Inputs=+-  SaturateOnIntegerOverflow=on  InputSameDT=on  OutDataTypeStr=Inherit: Same as first input
  Sum1 : Sum  Inputs=+++  SaturateOnIntegerOverflow=on  InputSameDT=on  OutDataTypeStr=Inherit: Same as first input
  Sum2 : Sum  SaturateOnIntegerOverflow=on  InputSameDT=on  OutDataTypeStr=Inherit: Same as first input
  Switch : Switch  Criteria=u2 > Threshold  SaturateOnIntegerOverflow=on  InputSameDT=on
  Switch1 : Switch  Criteria=u2 ~= 0  SaturateOnIntegerOverflow=on  InputSameDT=on
  Velocity : Outport
  Bus Out : Outport  Port=2
  wires:
  Sum1/1 -> Sum/2
  Tractive Force/1 -> Sum/1
  Aerodynamic Drag Function/1 -> Sum1/1
  Integrator1/1 -> [chs_plt_pos]
  Constant3/1 -> Switch/3
  Sum/1 -> Product/2
  Integrator/1 -> Saturation/1
  Switch/1 -> Sum1/3
  Constant5/1 -> Percent Grade to Radians/1
  Percent Grade to Radians/1 -> Rolling Resistance Function/1, Grade Resistance Function/1
  Product/1 -> Integrator/1
  Saturation/1 -> Memory/1, Velocity/1, [chs_plt_vel], Integrator1/1, Switch/2, Aerodynamic Drag Function/1
  Accelerator Position/1 -> Memory1/1  "Accelerator Position"
  Sum2/1 -> Switch1/2
  Switch1/1 -> Integrator/2
  Constant1/1 -> Switch1/1
  Constant2/1 -> Switch1/3
  Memory1/1 -> Sum2/2
  Memory/1 -> Sum2/1
  Constant6/1 -> Product/3
  Grade Resistance Function/1 -> Product1/1
  Product1/1 -> Sum1/2
  Constant4/1 -> Product1/2
  Constant/1 -> Product2/2
  Rolling Resistance Function/1 -> Product2/1
  Product2/1 -> Switch/1
  [chs_plt_vel] -> Bus Creator/1  "chs_plt_vel"
  [chs_plt_pos] -> Bus Creator/2  "chs_plt_pos"
  Bus Creator/1 -> Bus Out/1

== system EcoCAR3_Capstone_P2_LEA_GKN_Enerdel_TheREALone/Architecture/ESS/Plant ==
  Current : Inport
  1/num_cell_par : Gain  Gain=1/num_cell_par
  1/num_cell_par1 : Gain  Gain=1/num_cell_par
  Bus Creator : BusCreator
  SOC Calculation : Subsystem
  Voltage Calculation : Subsystem
  num_cell_series : Gain  Gain=num_cell_series
  num_cell_series1 : Gain  Gain=num_cell_series
  num_cell_series2 : Gain  Gain=num_cell_series
  "SOC " : Outport
  voltage : Outport  Port=2
  bus out : Outport  Port=3
  wires:
  Current/1 -> 1/num_cell_par/1
  SOC Calculation/1(SOC) -> Voltage Calculation/1(SOC), "SOC "/1
  1/num_cell_par/1 -> Voltage Calculation/2(Current), Bus Creator/4, SOC Calculation/1(Current)  "Current"
  Voltage Calculation/1(Open Circuit Voltage) -> num_cell_series/1
  Voltage Calculation/2(Voltage) -> num_cell_series1/1
  num_cell_series1/1 -> Bus Creator/2, voltage/1  "voltage"
  num_cell_series/1 -> Bus Creator/1  "voc"
  Voltage Calculation/3(Internal Resistance) -> num_cell_series2/1
  num_cell_series2/1 -> 1/num_cell_par1/1
  1/num_cell_par1/1 -> Bus Creator/3  "rint"
  Bus Creator/1 -> bus out/1

== system EcoCAR3_Capstone_P2_LEA_GKN_Enerdel_TheREALone/Architecture/ESS/ess_controller_PI ==
  In1 : Inport
  Bus Selector : BusSelector  OutputSignals=current,voltage,soc
  Controller : Subsystem
  Controller1 : Subsystem
  power_max_prop : Outport
  current_max_prop : Outport  Port=2
  power_max_reg : Outport  Port=3
  current_max_reg : Outport  Port=4
  wires:
  Bus Selector/3 -> Controller/3(SOC), Controller1/3(SOC)  "<soc>"
  Bus Selector/2 -> Controller/2(Voltage), Controller1/2(Voltage)  "<voltage>"
  Bus Selector/1 -> Controller1/1(Current), Controller1/4(Current1), Controller/4(Current1), Controller/1(Current)  "<current>"
  In1/1 -> Bus Selector/1
  Controller1/1(power_max_reg) -> power_max_reg/1  "power_max_reg"
  Controller/2(current_max_prop) -> current_max_prop/1  "current_max_prop"
  Controller1/2(current_max_reg) -> current_max_reg/1  "current_max_reg"
  Controller/1(power_max_prop) -> power_max_prop/1  "power_max_prop"

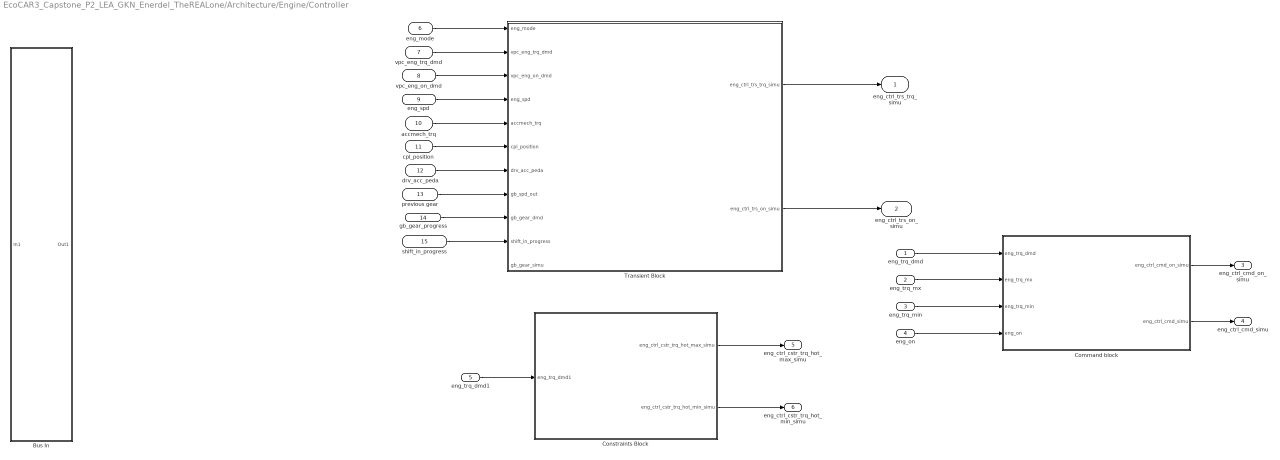
== system EcoCAR3_Capstone_P2_LEA_GKN_Enerdel_TheREALone/Architecture/Engine/Controller ==
  eng_trq_dmd : Inport
  eng_trq_mx : Inport  Port=2
  eng_trq_min : Inport  Port=3
  eng_on : Inport  Port=4
  eng_trq_dmd1 : Inport  Port=5
  eng_mode : Inport  Port=6
  vpc_eng_trq_dmd : Inport  Port=7
  vpc_eng_on_dmd : Inport  Port=8
  eng_spd : Inport  Port=9
  accmech_trq : Inport  Port=10
  cpl_position : Inport  Port=11
  drv_acc_peda : Inport  Port=12
  previous gear : Inport  Port=13
  gb_gear_progress : Inport  Port=14
  shift_in_progress : Inport  Port=15
  Bus In : Subsystem
  "Command block " : Subsystem
  Constraints Block : Subsystem
  Transient Block : Subsystem
  eng_ctrl_trs_trq_simu : Outport
  eng_ctrl_trs_on_simu : Outport  Port=2
  eng_ctrl_cmd_on_simu : Outport  Port=3
  eng_ctrl_cmd_simu : Outport  Port=4
  eng_ctrl_cstr_trq_hot_max_simu : Outport  Port=5
  eng_ctrl_cstr_trq_hot_min_simu : Outport  Port=6
  wires:
  eng_trq_dmd1/1 -> Constraints Block/1(eng_trq_dmd1)
  Constraints Block/1(eng_ctrl_cstr_trq_hot_max_simu) -> eng_ctrl_cstr_trq_hot_max_simu/1
  Constraints Block/2(eng_ctrl_cstr_trq_hot_min_simu) -> eng_ctrl_cstr_trq_hot_min_simu/1
  eng_trq_dmd/1 -> "Command block "/1(eng_trq_dmd)
  eng_trq_mx/1 -> "Command block "/2(eng_trq_mx)
  eng_trq_min/1 -> "Command block "/3(eng_trq_min)
  eng_on/1 -> "Command block "/4(eng_on)
  "Command block "/1(eng_ctrl_cmd_on_simu) -> eng_ctrl_cmd_on_simu/1
  "Command block "/2(eng_ctrl_cmd_simu) -> eng_ctrl_cmd_simu/1
  eng_mode/1 -> Transient Block/1(eng_mode)
  vpc_eng_trq_dmd/1 -> Transient Block/2(vpc_eng_trq_dmd)
  vpc_eng_on_dmd/1 -> Transient Block/3(vpc_eng_on_dmd)
  eng_spd/1 -> Transient Block/4(eng_spd)
  accmech_trq/1 -> Transient Block/5(accmech_trq)
  cpl_position/1 -> Transient Block/6(cpl_position)
  drv_acc_peda/1 -> Transient Block/7(drv_acc_peda)
  previous gear/1 -> Transient Block/8(gb_spd_out)
  shift_in_progress/1 -> Transient Block/10(shift_in_progress)
  Transient Block/1(eng_ctrl_trs_trq_simu) -> eng_ctrl_trs_trq_simu/1
  Transient Block/2(eng_ctrl_trs_on_simu) -> eng_ctrl_trs_on_simu/1
  gb_gear_progress/1 -> Transient Block/9(gb_gear_dmd)

== system EcoCAR3_Capstone_P2_LEA_GKN_Enerdel_TheREALone/Architecture/Engine/Plant1 ==
  Engine Speed : Inport
  Torque CMD % : Inport  Port=2
  Engine ON : Inport  Port=3
  Bus Creator : BusCreator
  Chart : Stateflow chart  TreatAsAtomicUnit=on
  Chart1 : Stateflow chart  TreatAsAtomicUnit=on
  Constant : Constant  Value=eng.plant.init.spd_str
  Fuel Rate Calc : Lookup_n-D  BreakpointsForDimension1=[1:3]  BreakpointsForDimension2=[1:3]  InternalRulePriority=Speed  RndMeth=Simplest  InputSameDT=on
  Integrator : Integrator
  Max WOT Torque : Lookup_n-D  NumberOfTableDimensions=1  BreakpointsForDimension1=engine.speed  Table=engine.torque  ExtrapMethod=Clip  DiagnosticForOutOfRangeInput=Warning  InternalRulePriority=Speed  RndMeth=Simplest  InputSameDT=on
  Relational Operator : RelationalOperator  OutDataTypeStr=boolean
  Stop Simulation : Stop
  eng.plant.mass.fuel : Constant
  engine off torque : Lookup_n-D  NumberOfTableDimensions=1  BreakpointsForDimension1=engine.speed  Table=engine.torque  ExtrapMethod=Clip  DiagnosticForOutOfRangeInput=Warning  InternalRulePriority=Speed  RndMeth=Simplest  InputSameDT=on
  min CTT torque : Lookup_n-D  NumberOfTableDimensions=1  BreakpointsForDimension1=engine.speed  Table=engine.torque  ExtrapMethod=Clip  DiagnosticForOutOfRangeInput=Warning  InternalRulePriority=Speed  RndMeth=Simplest  InputSameDT=on
  Bus Out : Outport
  Torque Out : Outport  Port=2
  wires:
  Max WOT Torque/1 -> Chart/4(max_eng_trq)
  Engine ON/1 -> Chart1/2(eng_on), Chart/1(eng_on)
  Torque CMD %/1 -> Chart/3(trq_cmd)
  engine off torque/1 -> Chart/6(eng_trq_eng_off)
  min CTT torque/1 -> Chart/5(min_eng_trq)
  Engine Speed/1 -> Chart1/4(eng_spd), Bus Creator/4, engine off torque/1, Fuel Rate Calc/2, min CTT torque/1, Max WOT Torque/1, Chart/2(eng_spd)  "eng_plnt_spd"
  Chart/1(eng_trq_out) -> Fuel Rate Calc/1, Bus Creator/1, Torque Out/1  "eng_plnt_trq_out"
  Fuel Rate Calc/1 -> Chart1/1(fuel_rate_in)
  Constant/1 -> Chart1/3(stalll_spd), Chart/7(stall_spd)
  Chart1/1(fuel_rate_out) -> Integrator/1, Bus Creator/2  "eng_plnt_fuel_rate"
  Integrator/1 -> Bus Creator/3, Relational Operator/1  "eng_plnt_fuel_cum"
  eng.plant.mass.fuel/1 -> Relational Operator/2
  Relational Operator/1 -> Stop Simulation/1
  Bus Creator/1 -> Bus Out/1

== system EcoCAR3_Capstone_P2_LEA_GKN_Enerdel_TheREALone/Architecture/Final Drive/Plant ==
  FD SPD Out : Inport
  FD Torque In : Inport  Port=2
  Divide : Product  Inputs=**
  "Final Drive Eff. " : Constant
  Final Drive Ratio : Constant
  Product : Product
  Product1 : Product
  SPD In : Outport
  Torque Out : Outport  Port=2
  wires:
  Final Drive Ratio/1 -> Divide/2, Product/2
  FD Torque In/1 -> Product/1
  Product/1 -> Product1/1
  "Final Drive Eff. "/1 -> Product1/2
  FD SPD Out/1 -> Divide/1
  Divide/1 -> SPD In/1
  Product1/1 -> Torque Out/1

== system EcoCAR3_Capstone_P2_LEA_GKN_Enerdel_TheREALone/Architecture/Gearbox/Controller ==
  In1 : Inport
  Bus Creator2 : BusCreator  Inputs=2
  Demand : Subsystem
  Transient : Subsystem
  Out1 : Outport
  wires:
  Demand/1(gb_ctrl_dmd_gear_simu) -> ?
  Transient/1(bus out) -> Bus Creator2/1  "transient"
  Demand/2(bus out) -> Bus Creator2/2  "demand"
  Bus Creator2/1 -> [CTRL]

== system EcoCAR3_Capstone_P2_LEA_GKN_Enerdel_TheREALone/Architecture/Gearbox/Plant ==
  GB SPD Out : Inport
  GB Torque in : Inport  Port=2
  Gear CMD : Inport  Port=3
  Divide : Product  Inputs=**
  Gear Efficiency Lookup : Lookup_n-D  NumberOfTableDimensions=1  BreakpointsForDimension1=[-5:5]  Table=tanh([-5:5])  InternalRulePriority=Speed  RndMeth=Simplest  InputSameDT=on
  Gear Ratio Lookup : Lookup_n-D  NumberOfTableDimensions=1  BreakpointsForDimension1=[-5:5]  Table=tanh([-5:5])  InternalRulePriority=Speed  RndMeth=Simplest  InputSameDT=on
  Product : Product
  Product1 : Product
  GB SPD In : Outport
  GB Torque Out : Outport  Port=2
  wires:
  Gear CMD/1 -> Gear Efficiency Lookup/1, Gear Ratio Lookup/1
  Gear Ratio Lookup/1 -> Divide/2, Product/2
  GB Torque in/1 -> Product/1
  GB SPD Out/1 -> Divide/1
  Product/1 -> Product1/1
  Gear Efficiency Lookup/1 -> Product1/2
  Product1/1 -> GB Torque Out/1
  Divide/1 -> GB SPD In/1

== system EcoCAR3_Capstone_P2_LEA_GKN_Enerdel_TheREALone/Architecture/Motor/Controller ==
  In1 : Inport
  Motor Controller : Subsystem
  Out1 : Outport
  bus out : Outport  Port=2

== system EcoCAR3_Capstone_P2_LEA_GKN_Enerdel_TheREALone/Architecture/Motor/Plant ==
  Motor Speed : Inport
  Torque CMD % : Inport  Port=2
  voltage : Inport  Port=3
  Bus Creator : BusCreator  Inputs=2
  Motor : Subsystem
  Torque Out : Outport
  Current : Outport  Port=2
  motor_plnt : Outport  Port=3
  wires:
  Motor Speed/1 -> Motor/1(Motor Speed)  "Motor Speed"
  Torque CMD %/1 -> Motor/2(Torque CMD %)
  Motor/1(Torque out) -> Bus Creator/1, Torque Out/1  "motor_plant_torque"
  Motor/2(Current) -> Bus Creator/2, Current/1  "motor_plant_current"
  voltage/1 -> Motor/3(Voltage)
  Bus Creator/1 -> motor_plnt/1

== system EcoCAR3_Capstone_P2_LEA_GKN_Enerdel_TheREALone/Architecture/Wheels/Plant ==
  Wheel Torque : Inport
  Linear Speed in : Inport  Port=2
  Constant : Constant
  Divide : Product  Inputs=*/
  Divide1 : Product  Inputs=*/
  Tractive Force : Outport
  Angular Speed : Outport  Port=2
  wires:
  Divide1/1 -> Angular Speed/1
  Linear Speed in/1 -> Divide1/1
  Wheel Torque/1 -> Divide/1
  Divide/1 -> Tractive Force/1
  Constant/1 -> Divide1/2, Divide/2

== system EcoCAR3_Capstone_P2_LEA_GKN_Enerdel_TheREALone/DriverControls/Velocity Profile/DriveCycle Select ==
  Cruise Test : FromWorkspace  VariableName=[CruiseTest.Time CruiseTest.SpdKph]  OutDataTypeStr=double  SampleTime=0
  FTP75 : FromWorkspace  VariableName=[UrbanCycle4.time(ftp75startind:end)-UrbanCycle4.time(ftp75startind) UrbanCycle4.SpdKph(ftp75startind:end)]  SampleTime=0
  HWY : FromWorkspace  VariableName=[EC_hwy.time EC_hwy.SpdKph]  SampleTime=0
  Multiport Switch : MultiPortSwitch  Inputs=6
  Select Cycle : Constant  Value=Drive_Cycle_Num
  US06 : FromWorkspace  VariableName=UrbanCycle6Rep  SampleTime=0.01  Interpolate=off  OutputAfterFinalValue=Cyclic repetition
  city 2 : FromWorkspace  VariableName=[EC_city2.time EC_city2.SpdKph]  SampleTime=0
  city1 : FromWorkspace  VariableName=[EC_city.time EC_city.SpdKph]  SampleTime=0
  kph : Outport
  wires:
  HWY/1 -> Multiport Switch/4
  Select Cycle/1 -> Multiport Switch/1
  city 2/1 -> Multiport Switch/3
  city1/1 -> Multiport Switch/2
  FTP75/1 -> Multiport Switch/5
  Multiport Switch/1 -> kph/1
  Cruise Test/1 -> Multiport Switch/6
  US06/1 -> Multiport Switch/7

== system EcoCAR3_Capstone_P2_LEA_GKN_Enerdel_TheREALone/DriverControls/Velocity Profile/Subsystem ==
  In1 : Inport
  In2 : Inport  Port=2
  In3 : Inport  Port=3
  Multiport Switch : MultiPortSwitch
  Select Mode : Constant  Value=Choice
  Out1 : Outport
  wires:
  In1/1 -> Multiport Switch/2
  Select Mode/1 -> Multiport Switch/1
  In3/1 -> Multiport Switch/4
  In2/1 -> Multiport Switch/3
  Multiport Switch/1 -> Out1/1

== system EcoCAR3_Capstone_P2_LEA_GKN_Enerdel_TheREALone/Supervisory Controller/Brake/Brake ECU Torque ==
  whl_trq_dmd : Inport
  1-D Lookup Table : Lookup_n-D  NumberOfTableDimensions=1  BreakpointsForDimension1=[-5:5]  Table=tanh([-5:5])  InternalRulePriority=Speed  RndMeth=Simplest  InputSameDT=on
  Abs : Abs
  Add : Sum  Inputs=+-
  Divide : Product  Inputs=/*
  Divider : Subsystem
  Fcn : Fcn  Expr=u<0
  Product : Product  Inputs=3
  Saturation : Saturate
  Transfer Fcn : TransferFcn  Denominator=[vpc.brake.init.time_cst_drv_trq_filter 1]
  mass_total : Constant  Value=veh_plant_init
  radius : Constant  Value=whl_plant_init
  whl_twr_brk_emergency : Outport
  whl_twr_brk_ECU : Outport  Port=2
  wires:
  Saturation/1 -> Add/1, Transfer Fcn/1
  Abs/1 -> Divide/2
  mass_total/1 -> Divider/2(In2)
  radius/1 -> Divide/1
  Product/1 -> Saturation/1
  Divide/1 -> Divider/1(In1)
  Divider/1(Out1) -> 1-D Lookup Table/1
  whl_trq_dmd/1 -> Product/1, Add/2, Abs/1, Fcn/1
  Transfer Fcn/1 -> whl_twr_brk_ECU/1
  Add/1 -> whl_twr_brk_emergency/1
  Fcn/1 -> Product/2
  1-D Lookup Table/1 -> Product/3

== system EcoCAR3_Capstone_P2_LEA_GKN_Enerdel_TheREALone/Supervisory Controller/Brake/Chassis speed ESS SOC limits ==
  whl_trq_brake_ECU : Inport
  chas_spd : Inport  Port=2
  ess_soc : Inport  Port=3
  Continuous Relay : Subsystem  mask(Continuous Relay){X_on=vpc.brake.init.ess_soc_above_regen_forbidden, X_off=vpc.brake.init.ess_soc_below_regen_allowed, Y_on=0, Y_off=1, ratio_trs=0.7}
      mask prompts: X_on "Switch on point"; X_off "Switch off point (must be lower than switch on point)"; Y_on "Output when on"; Y_off "Output when off"; ratio_trs "Transition Ratio (Between 0 and 1)"
      mask help: Works similarly to the original Matlab relay block. The transition between ON and OFF is continuous, and varies linearly
      mask init:
      | if X_on<=X_off
      |     error('Switch on point must be greater than switch off point')
      | end
      | 
      | if Y_on==Y_off
      |     error('ON and OFF values must be different')
      | end
      | 
      | if ratio_trs>1
      |     error('Transition ratio must be between 0 and 1')
      | end
      mask Display:
      | plot([0 0.2 0.4 1],[0.1 0.1 0.9 0.9])
      | plot([0 0.6 0.8 1],[0.1 0.1 0.9 0.9])
      | plot([0.5 0.5 ],[1.1 -0.1])
      | plot([-0.1 1.1 ],[0.5 0.5])
  Mechanical Regen Blending : Subsystem
  Product : Product  Inputs=3
  whl_trq_regen_available : Outport
  wires:
  whl_trq_brake_ECU/1 -> Product/3
  Mechanical Regen Blending/1(blend_factor) -> Product/2
  chas_spd/1 -> Mechanical Regen Blending/1(chas_spd)
  ess_soc/1 -> Continuous Relay/1(X)
  Product/1 -> whl_trq_regen_available/1
  Continuous Relay/1(Y) -> Product/1

== system EcoCAR3_Capstone_P2_LEA_GKN_Enerdel_TheREALone/Supervisory Controller/Brake/Electric power available ==
  ess_pwr_max_neg : Inport
  Divide : Product  Inputs=/*
  Divide1 : Product  Commented=on  Inputs=/*
  Sum1 : Sum  Inputs=+-
  eff_accelec_to_mot : Constant  Commented=on  Value=vpc_brake_init
  eff_ess_to_mot : Constant  Value=vpc_brake_init
  pwr_elec_available_regen : Outport
  wires:
  ? -> Divide1/2
  Sum1/1 -> pwr_elec_available_regen/1
  eff_ess_to_mot/1 -> Divide/1
  ess_pwr_max_neg/1 -> Divide/2
  eff_accelec_to_mot/1 -> Divide1/1
  Divide/1 -> Sum1/1

== system EcoCAR3_Capstone_P2_LEA_GKN_Enerdel_TheREALone/Supervisory Controller/Brake/Gear shifting ==
  gb_gear_ratio : Inport
  gb_sft_in_progress : Inport  Port=2
  cpl_cmd : Inport  Port=3
  Constant : Constant
  Constant1 : Constant
  Constant2 : Constant
  Constant3 : Constant  Value=0
  Memory : Memory
  Product : Product  Inputs=3
  Smooth Step Transition : Subsystem  mask(Smooth Transition for Steps){tau=vpc.brake.init.time_trs_sft}
      mask prompts: tau "Time constant"
      mask help:
      | Filters discontinuous first input, so that a smooth transition is created between the two values on each side of the discontinuity. Use to smooth a step (e.g. 0-1). Based on the 5-95%% output of a first order filter.
      | Second and Third inputs are the values on each side of the discontinuities, the highest value first.
      mask Display:
      | port_label('input',1,'x')
      | port_label('input',2,'max')
      | port_label('input',3,'min')
      | plot([0.2 0.4:0.1:0.9],0.8*[0 1-exp( 20*(0.4-[0.4:0.1:0.9]))]+0.1)
  Sum1 : Sum  Inputs=+-
  Switch : Switch  Criteria=u2 > Threshold  Threshold=0.5
  Switch1 : Switch  Criteria=u2 > Threshold
  cmd_cut_regen_cpl_open : Constant  Value=vpc_brake_init
  ratio_first_gear : Fcn  Expr=vpc_brake_init
  ratio_first_gear1 : Fcn  Expr=u>0
  ratio_first_gear2 : Fcn  Expr=u==1
  gear_ratio : Outport
  coeff_mult_gear : Outport  Port=2
  wires:
  cmd_cut_regen_cpl_open/1 -> Switch/2
  Constant1/1 -> Switch/3
  gb_gear_ratio/1 -> Switch1/1, Switch1/2, ratio_first_gear1/1
  Memory/1 -> ratio_first_gear/1
  Switch/1 -> ratio_first_gear2/1
  Product/1 -> coeff_mult_gear/1
  Constant3/1 -> Smooth Step Transition/3(X_min)
  ratio_first_gear/1 -> Switch1/3
  Constant/1 -> Sum1/1
  ratio_first_gear2/1 -> Product/2
  Constant2/1 -> Smooth Step Transition/2(X_max)
  ratio_first_gear1/1 -> Product/1
  gb_sft_in_progress/1 -> Sum1/2
  Switch1/1 -> gear_ratio/1, Memory/1
  cpl_cmd/1 -> Switch/1
  Smooth Step Transition/1(Out1) -> Product/3
  Sum1/1 -> Smooth Step Transition/1(X)

== system EcoCAR3_Capstone_P2_LEA_GKN_Enerdel_TheREALone/Supervisory Controller/Brake/Main motor brake torque demand ==
  whl_trq_regen_max : Inport
  ratio_gear : Inport  Port=2
  coef_mult_sft : Inport  Port=3
  mot_spd : Inport  Port=4
  mot_trq_max_regen : Inport  Port=5
  Divide : Product  Inputs=*/*
  Divide1 : Product  Inputs=/**
  Main motor electric power : Lookup_n-D  BreakpointsForDimension1=[1:3]  BreakpointsForDimension2=[1:3]  InternalRulePriority=Speed  RndMeth=Simplest  InputSameDT=on
  MinMax : MinMax  Function=max  Inputs=2
  Product : Product
  Product1 : Product
  mot_main_ratio_cum : Constant  Value=vpc_brake_init
  mot_main_reff_to_whl : Constant  Value=vpc_brake_init
  mot_trq_dmd : Outport
  mot_trq_dmd_at_wheels : Outport  Port=2
  mot_pwr_elec_estimated : Outport  Port=3
  wires:
  mot_main_reff_to_whl/1 -> Divide/2, Divide1/2
  mot_main_ratio_cum/1 -> Product/2
  mot_spd/1 -> Main motor electric power/1
  mot_trq_max_regen/1 -> Divide/3
  Main motor electric power/1 -> mot_pwr_elec_estimated/1
  MinMax/1 -> Product1/1
  whl_trq_regen_max/1 -> MinMax/2
  Product/1 -> Divide/1, Divide1/1
  Product1/1 -> mot_trq_dmd_at_wheels/1, Divide1/3
  coef_mult_sft/1 -> Product1/2
  Divide/1 -> MinMax/1
  ratio_gear/1 -> Product/1
  Divide1/1 -> mot_trq_dmd/1, Main motor electric power/2

== system EcoCAR3_Capstone_P2_LEA_GKN_Enerdel_TheREALone/Supervisory Controller/Brake/Motor main torque max ==
  mot_spd : Inport
  pwr_elec_max : Inport  Port=2
  mot_trq_max : Inport  Port=3
  Main motor power to torque : Lookup_n-D  BreakpointsForDimension1=[1:3]  BreakpointsForDimension2=[1:3]  InternalRulePriority=Speed  RndMeth=Simplest  InputSameDT=on
  MinMax : MinMax  Function=max  Inputs=2
  Saturation1 : Saturate  LowerLimit=-inf
  Saturation2 : Saturate  UpperLimit=0  LowerLimit=-inf
  mot_trq_maximum : Outport
  wires:
  pwr_elec_max/1 -> Main motor power to torque/2
  mot_spd/1 -> Main motor power to torque/1
  mot_trq_max/1 -> Saturation2/1
  Saturation1/1 -> MinMax/1
  Saturation2/1 -> MinMax/2
  Main motor power to torque/1 -> Saturation1/1
  MinMax/1 -> mot_trq_maximum/1

== system EcoCAR3_Capstone_P2_LEA_GKN_Enerdel_TheREALone/Supervisory Controller/Brake/Torque demand at wheels  ==
  brake_signal_dmd : Inport
  Pedal position to braking torque : Lookup_n-D  NumberOfTableDimensions=1  BreakpointsForDimension1=[-5:5]  Table=tanh([-5:5])  InternalRulePriority=Speed  RndMeth=Simplest  InputSameDT=on
  Saturation : Saturate  UpperLimit=0  LowerLimit=-inf
  whl_trq_dmd : Outport
  wires:
  brake_signal_dmd/1 -> Pedal position to braking torque/1
  Pedal position to braking torque/1 -> Saturation/1
  Saturation/1 -> whl_trq_dmd/1
